simulink model "regulator"  (R2018b)
settings: Solver=VariableStepAuto  StartTime=0.0  StopTime=10.0  RelTol=1e-3
values from neighbouring files (symbols this model uses):
  alfa = 0.01    [dane.m]
  beta = 0.1    [dane.m]
  k = 400    [dane.m]
settings Model: Creator=lpa1  LastModifiedBy=Sonia

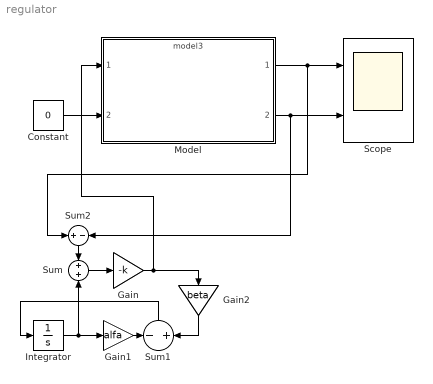
== system regulator ==
  Constant : Constant  Value=0
  Gain : Gain  Gain=-k
  Gain1 : Gain  Gain=alfa
  Gain2 : Gain  Gain=beta
  Integrator : Integrator  InitialCondition=1
  Model : ModelReference  ModelNameDialog=model3.slx  SimulationMode=Normal  ModelReferenceVersion=1.10
  Scope : Scope  NumInputPorts=2
  Sum : Sum
  Sum1 : Sum  Inputs=-+
  Sum2 : Sum  Inputs=+-
  wires:
  Constant/1 -> Model/2
  Model/2 -> Scope/2, Sum2/2
  Model/1 -> Sum2/1, Scope/1
  Sum/1 -> Gain/1
  Integrator/1 -> Gain1/1, Sum/2
  Sum1/1 -> Integrator/1
  Sum2/1 -> Sum/1
  Gain/1 -> Gain2/1, Model/1
  Gain1/1 -> Sum1/1
  Gain2/1 -> Sum1/2
